simulink model "servo_control_cube_operations_test"  (R2022b)
settings: Solver=FixedStepDiscrete  StartTime=0.0  StopTime=10.0  RelTol=1e-3
InitFcn:
  | mbd_s32k_consistency_checks(bdroot(gcs));
undefined symbols (not defined in the file or in its folder): LQFP
libraries: mbd_s32k1xx_ec_toolbox x3
settings Model: Creator=leona  LastModifiedBy=leona
settings DataIOCC: ExternalInput=off  InitialState=off  SaveOutput=off  SaveState=on  SaveTime=off
settings OptimizationCC: DefaultParameterBehavior=Inlined  EnhancedBackFolding=on  PassReuseOutputArgsAs=Individual arguments  ZeroExternalMemoryAtStartup=off  ZeroInternalMemoryAtStartup=off  OptimizeBlockOrder=speed  DifferentSizesBufferReuse=on  OptimizationCustomize=off  EfficientTunableParamExpr=on
settings DebuggingCC: InheritedTsInSrcMsg=none  SingleTaskRateTransMsg=error  ParameterTunabilityLossMsg=error  UnconnectedInputMsg=error  UnconnectedOutputMsg=error  UnconnectedLineMsg=error  UnknownTsInhSupMsg=error
settings HardwareCC: ProdBitPerPointer=32  ProdBitPerSizeT=32  ProdBitPerPtrDiffT=32  ProdLargestAtomicInteger=Long  ProdLargestAtomicFloat=Double  ProdWordSize=32  ProdHWDeviceType=ARM Compatible->ARM Cortex
settings ModelReferenceCC: ModelReferenceNumInstancesAllowed=Single
settings SFSimCC: MATLABDynamicMemAlloc=off
settings RTWCC: Description=Model Based Design Toolbox S32K1xx Code Generation Target  SystemTargetFile=mbd_s32k.tlc  MakeCommand=mbd_s32k_make_rtw COPY_MDLREF_INCLUDES=0  TemplateMakefile=mbd_s32k.tmf
settings CodeAppCC: ForceParamTrailComments=on  IgnoreCustomStorageClasses=off  OperatorAnnotations=on  SimulinkDataObjDesc=on  SFDataObjDesc=on  InsertBlockDesc=on
settings STFCustomTargetCC: TargetLangStandard=C99 (ISO)  MultiwordLength=256  CombineOutputUpdateFcns=on  ERTCustomFileBanners=on  SupportContinuousTime=off  SupportNonInlinedSFcns=off  RemoveResetFunc=on  MATLABClassNameForMDSCustomization=Simulink.SoftwareTarget.ERTCustomization  SystemTargetFile=mbd_s32k.tlc
settings ERTTargetCC: TargetLangStandard=C99 (ISO)  ParMdlRefBuildCompliant=off  CompOptLevelCompliant=off  ConcurrentExecutionCompliant=off  ModelStepFunctionPrototypeControlCompliant=off  CPPClassGenCompliant=off  UseToolchainInfoCompliant=off  InlinedParameterPlacement=NonHierarchical  ERTSrcFileBannerTemplate=mbd_ert_code_template.cgt  ERTHdrFileBannerTemplate=mbd_ert_code_template.cgt  ERTDataSrcFileTemplate=mbd_ert_code_template.cgt  ERTDataHdrFileTemplate=mbd_ert_code_template.cgt  ERTCustomFileTemplate=example_file_process.tlc

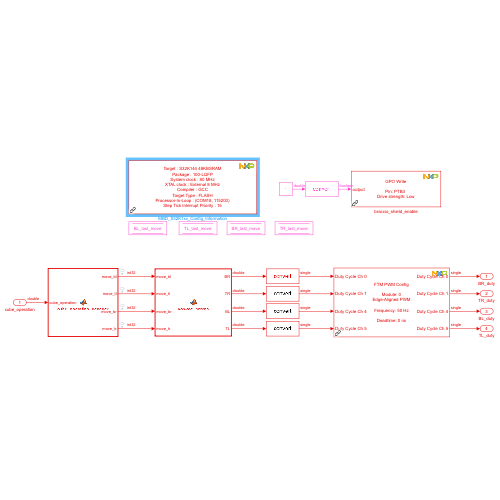
[thumbnail: Simulink's stored preview of the top-level diagram]
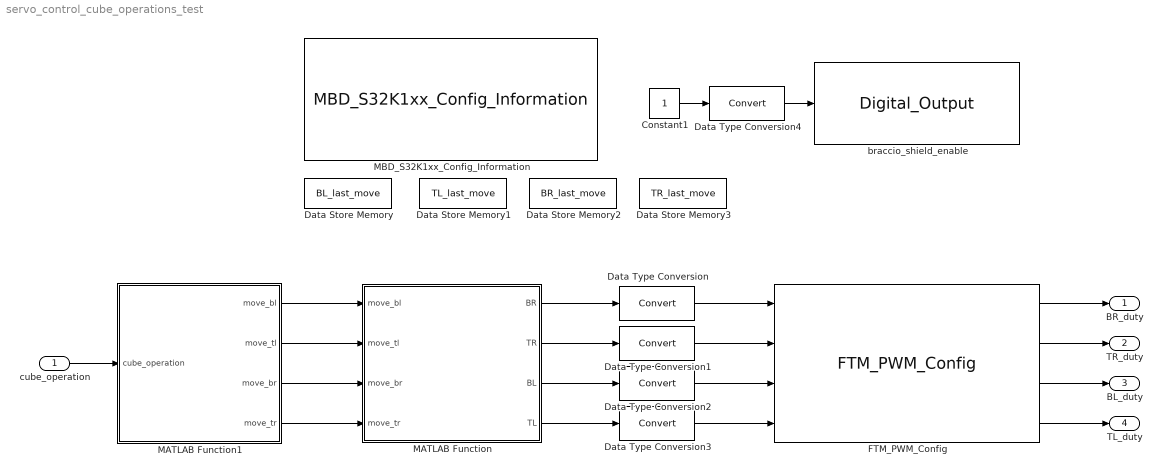
== system servo_control_cube_operations_test ==
  cube_operation : Inport
  Constant1 : Constant
  Data Store Memory : DataStoreMemory  DataStoreName=BL_last_move  WriteAfterWriteMsg=warning  ShowAdditionalParam=off
  Data Store Memory1 : DataStoreMemory  DataStoreName=TL_last_move  WriteAfterWriteMsg=warning  ShowAdditionalParam=off
  Data Store Memory2 : DataStoreMemory  DataStoreName=BR_last_move  WriteAfterWriteMsg=warning  ShowAdditionalParam=off
  Data Store Memory3 : DataStoreMemory  DataStoreName=TR_last_move  WriteAfterWriteMsg=warning  ShowAdditionalParam=off
  Data Type Conversion{,1..4} (5 alike) : DataTypeConversion  SaturateOnIntegerOverflow=off  RndMeth=Floor
  FTM_PWM_Config : mbd_s32k1xx_ec_toolbox/Motor Control Blocks/FTM Blocks/FTM_PWM_Config  ftmModule=0  ftmMode=Edge-Aligned PWM  ftmSourceClock=80 MHz  swcontrol_enable=off  chan0En=on  chan0Type=Independent  chan2En=off  chan2Type=Independent  chan4En=on  chan4Type=Independent  chan6En=off  chan6Type=Independent  ftmPwmUnits=Hz  outFrequency=50  ftmPeriod=25000  ftmPrescaler=Divide by 64  deadtimeUnits=Nanoseconds  deadtimeNs=0  deadtimeTicks=0  deadtimePrescaler=Divide by 1  dutyCycleCh0=0.03  dutyCycleCh1=0.125  dutyCycleCh2=0.025  dutyCycleCh3=0.025  dutyCycleCh4=0.025  dutyCycleCh5=0.025  dutyCycleCh6=0.25  dutyCycleCh7=0.25  dutyCycleSim=on  startAfterInit=on  showAdvOpt=on  pinFtmCh0=PTD15: [FTM0_CH0 | FTM Channel]  pinFtmCh1=PTD16: [FTM0_CH1 | FTM Channel]  pinPolCh0=Active High  pinPolCh1=Active High  outputComplem0=Main duplicated  outputLevel0=Low  outputLevel1=Low  pinFtmCh2=PTB14: [FTM0_CH2 | FTM Channel]  pinFtmCh3=PTC3: [FTM0_CH3 | FTM Channel]  pinPolCh2=Active High  pinPolCh3=Active High  outputComplem2=Main duplicated  outputLevel2=Low  outputLevel3=Low  pinFtmCh4=PTB4: [FTM0_CH4 | FTM Channel]  pinFtmCh5=PTB5: [FTM0_CH5 | FTM Channel]  pinPolCh4=Active High  pinPolCh5=Active High  outputComplem4=Main duplicated  outputLevel4=Low  outputLevel5=Low  pinFtmCh6=PTE8: [FTM0_CH6 | FTM Channel]  pinFtmCh7=None  pinPolCh6=Active High  pinPolCh7=Active High  outputComplem6=Main duplicated  outputLevel6=Low  outputLevel7=Low  initTrigger=off  chTrigger0=off  chTrigger1=off  chTrigger2=off  chTrigger3=off  chTrigger4=off  chTrigger5=off  chTrigger6=off  chTrigger7=off  mcuTargetUpdate=on  pwmSyncTrg=Software trigger  pwmSyncHwRouting=TRGMUX_FTM7  pwmSyncTrg0=off  pwmSyncTrg1=off  pwmSyncTrg2=off  pwmSyncAutoClear=on  pwmSyncMinLoad=on  pwmSyncMaxLoad=on  pwmSyncInvert=System Clock  pwmSyncOutControl=System Clock  pwmSyncOutMask=System Clock  pwmSyncCounterInitial=System Clock  pwmSyncPoints=Update now  reloadEnable=off  reloadPriority=15  reloadHalfCycle=off  reloadHCR=0  reloadFrequency=0  chnMatch0=off  chnMatch1=off  chnMatch2=off  chnMatch3=off  chnMatch4=off  chnMatch5=off  chnMatch6=off  chnMatch7=off  pwmFaultProtection=off  pwmFaultInterrupt=off  pwmFaultClearing=Fault control disabled  pwmFaultPinState=Safe Value  pwmFaultFilterValue=0  pwmFaultPriority=15  fault_disen_0=off  fault_filter_0=off  fault_polarity_0=Active High  fault_disen_1=off  fault_filter_1=off  fault_polarity_1=Active high  fault_disen_2=off  fault_filter_2=off  fault_polarity_2=Active high  fault_disen_3=off  fault_filter_3=off  fault_polarity_3=Active high  fault_pin_0=None  fault_pin_1=None  fault_pin_2=None  fault_pin_3=None
  MATLAB Function : MATLAB Function  TreatAsAtomicUnit=on
  MATLAB Function1 : MATLAB Function  TreatAsAtomicUnit=on
  MBD_S32K1xx_Config_Information : mbd_s32k1xx_ec_toolbox/MBD_S32K1xx_Config_Information  mbdt_ver=0  disp_str=|  config_params=[]  mcu_target_name=S32K144  mcu_target_package=100-LQFP  mcu_target_sram_size=48KB  mcu_system_clock_freq=80  mcu_xtal_freq=External 8  mcu_steptick_timer=LPIT Channel 0  mcu_steptick_prio=15  ds_import_enable=on  target_compiler=GCC  target_memory=FLASH  gcc_target_compile_opts=-mthumb -mfloat-abi=hard -mfpu=fpv4-sp-d16 -O1 -g -gstrict-dwarf  gcc_target_assemble_opts=-mthumb -mfloat-abi=hard -mfpu=fpv4-sp-d16 -g  gcc_target_link_opts=-mthumb -mfloat-abi=hard -mfpu=fpv4-sp-d16  gcc_target_default_lcf=on  gcc_target_user_lcf=S32K144_48_flash.ld  ghs_target_compile_opts=-cpu=cortexm4f -thumb -fpu=vfpv4_d16 -fsingle -Ogeneral -Wundef -Wimplicit-int -Wshadow -Wtrigraphs --no_commons --gnu_asm -gnu99 -gdwarf-2 -G  ghs_target_assemble_opts=-cpu=cortexm4f -fpu=vfpv4_d16  ghs_target_link_opts=-cpu=cortexm4f -thumb -fpu=vfpv4_d16  ghs_target_default_lcf=on  ghs_target_user_lcf=S32K144_48_flash.ld  iar_target_compile_opts=--cpu=Cortex-M4F --thumb --fpu=VFPv4_sp -Ol -e --debug --dlib_config normal  iar_target_assemble_opts=--cpu Cortex-M4F --thumb --fpu VFPv4_sp  iar_target_link_opts=--no_exceptions --vfe --inline  iar_target_default_lcf=on  iar_target_user_lcf=S32K144_48_flash.icf  pil_download_enable=on  rbl_download_enable=on  rbl_start_delay=5000  rbl_download_interface=OpenSDA  rbl_restart_request=off  rbl_com_port=Custom  rbl_com_port_custom=COM18  pil_download_rate=115200  pil_download_rate_custom=115200  pil_opensda_drive=F: EVB-S32K144  pil_opensda_drive_custom=D  jtag_interface=OpenSDA Embedded Debug  jlink_default_path=on  jlink_user_path=C:\Program Files\SEGGER\JLink\  pil_uart_instance=1  pil_uart_rx=PTC6: [LPUART1_RX | Receive]  pil_uart_tx=PTC7: [LPUART1_TX | Transmit]  FTM_PWM_PcrCheckEnDis=on  FTM_Input_Edge_Inputs_PcrCheckEnDis=on  FTM_Dual_Edge_Inputs_PcrCheckEnDis=on  FTM_Quadrature_Inputs_PcrCheckEnDis=on  FTM_Hall_Sensor_Inputs_PcrCheckEnDis=on  LPTMR_PcrCheckEnDis=on  PIT_PcrCheckEnDis=on  RTC_PcrCheckEnDis=on  FlexCAN_PcrCheckEnDis=on  LIN_PcrCheckEnDis=on  FlexIO_PcrCheckEnDis=on  LPI2C_PcrCheckEnDis=on  LPSPI_PcrCheckEnDis=on  LPUART_PcrCheckEnDis=on  CMP_PcrCheckEnDis=on  GPIO_OutputPcrCheckEnDis=on  GPIO_InputPcrCheckEnDis=on  SBC_PcrCheckEnDis=on  BMS_PcrCheckEnDis=on  AMMCLIB_PcrCheckEnDis=on  FM_PcrCheckEnDis=on  Profile_PcrCheckEnDis=on  ConfigParams_PcrCheckEnDis=on  ModelRef_PcrCheckEnDis=on  PDB0_PcrCheckEnDis=on  CSEc_PcrCheckEnDis=on  eDMA_PcrCheckEnDis=on  FLASH_PcrCheckEnDis=on  ADC_PcrCheckEnDis=on  WDOG_PcrCheckEnDis=on
      | Target : S32K144-64KB_SRAM
      | Package : 100-pin
      | System clock : 80 MHz
      | XTAL clock : External 8 MHz
      | Compiler : IAR
      | Target Type : FLASH
      | Download Code after build : off
      | Step Tick Interrupt Priority : 15
  braccio_shield_enable : mbd_s32k1xx_ec_toolbox/GPIO Blocks/Digital_Output  gpio_pin=PTB3: [PTB3 | Port B I/O]  init_val=Low  drive_strength=Low
  BR_duty : Outport
  TR_duty : Outport  Port=2
  BL_duty : Outport  Port=3
  TL_duty : Outport  Port=4
  wires:
  Data Type Conversion4/1 -> braccio_shield_enable/1
  Constant1/1 -> Data Type Conversion4/1
  MATLAB Function1/1(move_bl) -> MATLAB Function/1(move_bl)
  MATLAB Function1/2(move_tl) -> MATLAB Function/2(move_tl)
  MATLAB Function1/3(move_br) -> MATLAB Function/3(move_br)
  MATLAB Function1/4(move_tr) -> MATLAB Function/4(move_tr)
  cube_operation/1 -> MATLAB Function1/1(cube_operation)
  MATLAB Function/1(BR) -> Data Type Conversion/1
  MATLAB Function/2(TR) -> Data Type Conversion1/1
  MATLAB Function/4(TL) -> Data Type Conversion3/1
  MATLAB Function/3(BL) -> Data Type Conversion2/1
  Data Type Conversion3/1 -> FTM_PWM_Config/4
  FTM_PWM_Config/4 -> TL_duty/1
  FTM_PWM_Config/2 -> TR_duty/1
  FTM_PWM_Config/1 -> BR_duty/1
  Data Type Conversion/1 -> FTM_PWM_Config/1
  Data Type Conversion2/1 -> FTM_PWM_Config/3
  FTM_PWM_Config/3 -> BL_duty/1
  Data Type Conversion1/1 -> FTM_PWM_Config/2

== matlab function servo_control_cube_operations_test/MATLAB Function1 ==
  data: cube_operation input; move_bl output; move_tl output; move_br output; move_tr output
function [move_bl, move_tl, move_br, move_tr] = cube_operation_decoder(cube_operation)
% This function takes as input the code for a cube operation and converts
% it as positions of the 4 servo motors. The operations must be a 4 digit
% unsigned integer, encoded as follows:
%   - first digit [0, 1]: open/close left grip;
%   - second digit [0, 1]: open/close right grip;
%   - third digit [0, 1, 2]: set left arm to 90/0/180 degrees
%   - fourth digit [0, 1, 2]: set right arm to 90/0/180 degress

x1 = int32(mod(cube_operation/1000, 10));
x2 = int32(mod(cube_operation/100, 10));
x3 = int32(mod(cube_operation/10, 10));
x4 = int32(mod(cube_operation, 10));

move_tl = x1;
move_tr = x2;
move_bl = x3;
move_br = x4;

== matlab function servo_control_cube_operations_test/MATLAB Function ==
  data: BR output; TR output; move_bl input; BL output; move_tl input; move_br input; move_tr input; TL output
function [BR, TR, BL, TL] = actuate_servos(move_bl, move_tl, move_br, move_tr)
% This function takes as input as specific number associated to a movement
% of the 4 servo motors (BL = Bottom Left, TL = Top Left, BR = Bottom Right,
% TR = Top Right) and it gives as output the 4 relative duty cycles needed to
% obtain that movement. 

min_duty = 0.025;
max_duty = 0.125;

duty_0_deg = min_duty;
duty_grip_open = min_duty + (max_duty-min_duty)/3;
duty_grip_closed = min_duty + (max_duty-min_duty)/9; 
duty_90_deg = min_duty + (max_duty-min_duty)/2;
duty_180_deg = max_duty;

switch (move_tl)
    case 0                  % Open left grip
        TL = duty_grip_open;
    case 1                  % Close left grip
        TL = duty_grip_closed;
    otherwise               % Open left grip
        TL = duty_grip_open;
end

switch (move_tr)
    case 0                  % Open right grip
        TR = duty_grip_open;
    case 1                  % Close right grip
        TR = duty_grip_closed;
    otherwise               % Open right grip
        TR = duty_grip_open;
end

switch (move_bl)
    case 0                  % Left arm straight
        BL = duty_90_deg;
    case 1                  % Left arm at 90° clockwise
        BL = duty_0_deg;
    case 2                 % Left arm at 90° counter-clockwise
        BL = duty_180_deg;
    otherwise
        BL = duty_90_deg;
end

switch (move_br)
    case 0                  % Right arm straight
        BR = duty_90_deg;
    case 1                  % Right arm at 90° clockwise
        BR = duty_0_deg;
    case 2                 % Right arm at 90° counter-clockwise
        BR = duty_180_deg;
    otherwise
        BR = duty_90_deg;
end

% Update current position of the motors
BL_last_move = move_bl;
TL_last_move = move_tl;
BR_last_move = move_br;
TR_last_move = move_tr;
